simulink model "model"  (R2014a)
(part 4 of 4)

  L_186634762/LConn3 -- T_186634762__/RConn3 -- bus221/LConn1
  T_340152021__/RConn1 -- L_340152021/LConn1
  T_340152021__/RConn2 -- L_340152021/LConn2
  L_340152021/LConn3 -- T_340152021__/RConn3 -- bus222/LConn1
  T_265318415__/RConn1 -- L_265318415/LConn1
  T_265318415__/RConn2 -- L_265318415/LConn2
  L_265318415/LConn3 -- T_265318415__/RConn3 -- bus223/LConn1
  T_246972431__/RConn1 -- L_246972431/LConn1
  T_246972431__/RConn2 -- L_246972431/LConn2
  L_246972431/LConn3 -- T_246972431__/RConn3 -- bus224/LConn1
  T_234372891__/RConn1 -- L_234372891/LConn1
  T_234372891__/RConn2 -- L_234372891/LConn2
  L_234372891/LConn3 -- T_234372891__/RConn3 -- bus225/LConn1
  T_269492241__/RConn1 -- L_269492241/LConn1
  T_269492241__/RConn2 -- L_269492241/LConn2
  L_269492241/LConn3 -- T_269492241__/RConn3 -- bus226/LConn1
  T_160831508__/RConn1 -- L_160831508/LConn1
  T_160831508__/RConn2 -- L_160831508/LConn2
  L_160831508/LConn3 -- T_160831508__/RConn3 -- bus227/LConn1
  T_160831511__/RConn1 -- L_160831511/LConn1
  T_160831511__/RConn2 -- L_160831511/LConn2
  L_160831511/LConn3 -- T_160831511__/RConn3 -- bus228/LConn1
  T_399067566__/RConn1 -- L_399067566/LConn1
  T_399067566__/RConn2 -- L_399067566/LConn2
  L_399067566/LConn3 -- T_399067566__/RConn3 -- bus229/LConn1
  T_399067557__/RConn1 -- L_399067557/LConn1
  T_399067557__/RConn2 -- L_399067557/LConn2
  L_399067557/LConn3 -- T_399067557__/RConn3 -- bus230/LConn1
  T_167008794__/RConn1 -- L_167008794/LConn1
  T_167008794__/RConn2 -- L_167008794/LConn2
  L_167008794/LConn3 -- T_167008794__/RConn3 -- bus231/LConn1
  T_199476036__/RConn1 -- L_199476036/LConn1
  T_199476036__/RConn2 -- L_199476036/LConn2
  L_199476036/LConn3 -- T_199476036__/RConn3 -- bus232/LConn1
  T_311980589__Gardu_Induk_Alta_Prima/RConn1 -- L_311980589/LConn1
  T_311980589__Gardu_Induk_Alta_Prima/RConn2 -- L_311980589/LConn2
  L_311980589/LConn3 -- T_311980589__Gardu_Induk_Alta_Prima/RConn3 -- bus233/LConn1
  T_166644946__Gardu_Induk_Surabaya_Barat/RConn1 -- L_166644946/LConn1
  T_166644946__Gardu_Induk_Surabaya_Barat/RConn2 -- L_166644946/LConn2
  L_166644946/LConn3 -- T_166644946__Gardu_Induk_Surabaya_Barat/RConn3 -- bus234/LConn1
  T_277204741__/RConn1 -- L_277204741/LConn1
  T_277204741__/RConn2 -- L_277204741/LConn2
  L_277204741/LConn3 -- T_277204741__/RConn3 -- bus235/LConn1
  T_276990481__/RConn1 -- L_276990481/LConn1
  T_276990481__/RConn2 -- L_276990481/LConn2
  L_276990481/LConn3 -- T_276990481__/RConn3 -- bus236/LConn1
  T_228490272__Gardu_Induk_PLN_Palur/RConn1 -- L_228490272/LConn1
  T_228490272__Gardu_Induk_PLN_Palur/RConn2 -- L_228490272/LConn2
  L_228490272/LConn3 -- T_228490272__Gardu_Induk_PLN_Palur/RConn3 -- bus237/LConn1
  T_265030543__/RConn1 -- L_265030543/LConn1
  T_265030543__/RConn2 -- L_265030543/LConn2
  L_265030543/LConn3 -- T_265030543__/RConn3 -- bus238/LConn1
  T_268865917__/RConn1 -- L_268865917/LConn1
  T_268865917__/RConn2 -- L_268865917/LConn2
  L_268865917/LConn3 -- T_268865917__/RConn3 -- bus239/LConn1
  T_104412357__/RConn1 -- L_104412357/LConn1
  T_104412357__/RConn2 -- L_104412357/LConn2
  L_104412357/LConn3 -- T_104412357__/RConn3 -- bus240/LConn1
  T_311479841__Gardu_Sekar_Bungu/RConn1 -- L_311479841/LConn1
  T_311479841__Gardu_Sekar_Bungu/RConn2 -- L_311479841/LConn2
  L_311479841/LConn3 -- T_311479841__Gardu_Sekar_Bungu/RConn3 -- bus241/LConn1
  T_311666431__Gardu_Induk_Gili_Timur/RConn1 -- L_311666431/LConn1
  T_311666431__Gardu_Induk_Gili_Timur/RConn2 -- L_311666431/LConn2
  L_311666431/LConn3 -- T_311666431__Gardu_Induk_Gili_Timur/RConn3 -- bus242/LConn1
  T_311666430__Gardu_Induk_Bangkalan/RConn1 -- L_311666430/LConn1
  T_311666430__Gardu_Induk_Bangkalan/RConn2 -- L_311666430/LConn2
  L_311666430/LConn3 -- T_311666430__Gardu_Induk_Bangkalan/RConn3 -- bus243/LConn1
  T_398909637__/RConn1 -- L_398909637/LConn1
  T_398909637__/RConn2 -- L_398909637/LConn2
  L_398909637/LConn3 -- T_398909637__/RConn3 -- bus244/LConn1
  T_311485046__Gardu_Induk_Cerme/RConn1 -- L_311485046/LConn1
  T_311485046__Gardu_Induk_Cerme/RConn2 -- L_311485046/LConn2
  L_311485046/LConn3 -- T_311485046__Gardu_Induk_Cerme/RConn3 -- bus245/LConn1
  T_264855643__/RConn1 -- L_264855643/LConn1
  T_264855643__/RConn2 -- L_264855643/LConn2
  L_264855643/LConn3 -- T_264855643__/RConn3 -- bus246/LConn1
  T_265002737__/RConn1 -- L_265002737/LConn1
  T_265002737__/RConn2 -- L_265002737/LConn2
  L_265002737/LConn3 -- T_265002737__/RConn3 -- bus247/LConn1
  T_264855645__/RConn1 -- L_264855645/LConn1
  T_264855645__/RConn2 -- L_264855645/LConn2
  L_264855645/LConn3 -- T_264855645__/RConn3 -- bus248/LConn1
  T_248953893__/RConn1 -- L_248953893/LConn1
  T_248953893__/RConn2 -- L_248953893/LConn2
  L_248953893/LConn3 -- T_248953893__/RConn3 -- bus249/LConn1
  T_248953894__/RConn1 -- L_248953894/LConn1
  T_248953894__/RConn2 -- L_248953894/LConn2
  L_248953894/LConn3 -- T_248953894__/RConn3 -- bus250/LConn1
  T_267663602__/RConn1 -- L_267663602/LConn1
  T_267663602__/RConn2 -- L_267663602/LConn2
  L_267663602/LConn3 -- T_267663602__/RConn3 -- bus251/LConn1
  T_279284589__/RConn1 -- L_279284589/LConn1
  T_279284589__/RConn2 -- L_279284589/LConn2
  L_279284589/LConn3 -- T_279284589__/RConn3 -- bus252/LConn1
  T_195105324__/RConn1 -- L_195105324/LConn1
  T_195105324__/RConn2 -- L_195105324/LConn2
  L_195105324/LConn3 -- T_195105324__/RConn3 -- bus253/LConn1
  T_398925619__/RConn1 -- L_398925619/LConn1
  T_398925619__/RConn2 -- L_398925619/LConn2
  L_398925619/LConn3 -- T_398925619__/RConn3 -- bus254/LConn1
  T_195211467__/RConn1 -- L_195211467/LConn1
  T_195211467__/RConn2 -- L_195211467/LConn2
  L_195211467/LConn3 -- T_195211467__/RConn3 -- bus255/LConn1
  T_268846126__/RConn1 -- L_268846126/LConn1
  T_268846126__/RConn2 -- L_268846126/LConn2
  L_268846126/LConn3 -- T_268846126__/RConn3 -- bus256/LConn1
  T_268846115__/RConn1 -- L_268846115/LConn1
  T_268846115__/RConn2 -- L_268846115/LConn2
  L_268846115/LConn3 -- T_268846115__/RConn3 -- bus257/LConn1
  T_268831411__/RConn1 -- L_268831411/LConn1
  T_268831411__/RConn2 -- L_268831411/LConn2
  L_268831411/LConn3 -- T_268831411__/RConn3 -- bus258/LConn1
  T_399724591__/RConn1 -- L_399724591/LConn1
  T_399724591__/RConn2 -- L_399724591/LConn2
  L_399724591/LConn3 -- T_399724591__/RConn3 -- bus259/LConn1
  T_399724593__/RConn1 -- L_399724593/LConn1
  T_399724593__/RConn2 -- L_399724593/LConn2
  L_399724593/LConn3 -- T_399724593__/RConn3 -- bus260/LConn1
  T_162030133__/RConn1 -- L_162030133/LConn1
  T_162030133__/RConn2 -- L_162030133/LConn2
  L_162030133/LConn3 -- T_162030133__/RConn3 -- bus261/LConn1
  T_162030143__/RConn1 -- L_162030143/LConn1
  T_162030143__/RConn2 -- L_162030143/LConn2
  L_162030143/LConn3 -- T_162030143__/RConn3 -- bus262/LConn1
  T_162002076__/RConn1 -- L_162002076/LConn1
  T_162002076__/RConn2 -- L_162002076/LConn2
  L_162002076/LConn3 -- T_162002076__/RConn3 -- bus263/LConn1
  T_263932883__/RConn1 -- L_263932883/LConn1
  T_263932883__/RConn2 -- L_263932883/LConn2
  L_263932883/LConn3 -- T_263932883__/RConn3 -- bus264/LConn1
  T_311479840__Gardu_Induk_Segoromadu/RConn1 -- L_311479840/LConn1
  T_311479840__Gardu_Induk_Segoromadu/RConn2 -- L_311479840/LConn2
  L_311479840/LConn3 -- T_311479840__Gardu_Induk_Segoromadu/RConn3 -- bus265/LConn1
  T_311479839__Gardu_Induk_Petrokimia/RConn1 -- L_311479839/LConn1
  T_311479839__Gardu_Induk_Petrokimia/RConn2 -- L_311479839/LConn2
  L_311479839/LConn3 -- T_311479839__Gardu_Induk_Petrokimia/RConn3 -- bus266/LConn1
  T_398909625__/RConn1 -- L_398909625/LConn1
  T_398909625__/RConn2 -- L_398909625/LConn2
  L_398909625/LConn3 -- T_398909625__/RConn3 -- bus267/LConn1
  T_161951304__/RConn1 -- L_161951304/LConn1
  T_161951304__/RConn2 -- L_161951304/LConn2
  L_161951304/LConn3 -- T_161951304__/RConn3 -- bus268/LConn1
  T_399038176__/RConn1 -- L_399038176/LConn1
  T_399038176__/RConn2 -- L_399038176/LConn2
  L_399038176/LConn3 -- T_399038176__/RConn3 -- bus269/LConn1
  T_399038175__/RConn1 -- L_399038175/LConn1
  T_399038175__/RConn2 -- L_399038175/LConn2
  L_399038175/LConn3 -- T_399038175__/RConn3 -- bus270/LConn1
  T_161948635__/RConn1 -- L_161948635/LConn1
  T_161948635__/RConn2 -- L_161948635/LConn2
  L_161948635/LConn3 -- T_161948635__/RConn3 -- bus271/LConn1
  T_264713279__/RConn1 -- L_264713279/LConn1
  T_264713279__/RConn2 -- L_264713279/LConn2
  L_264713279/LConn3 -- T_264713279__/RConn3 -- bus272/LConn1
  T_269129296__/RConn1 -- L_269129296/LConn1
  T_269129296__/RConn2 -- L_269129296/LConn2
  L_269129296/LConn3 -- T_269129296__/RConn3 -- bus273/LConn1
  T_399067568__/RConn1 -- L_399067568/LConn1
  T_399067568__/RConn2 -- L_399067568/LConn2
  L_399067568/LConn3 -- T_399067568__/RConn3 -- bus274/LConn1
  T_265923575__/RConn1 -- L_265923575/LConn1
  T_265923575__/RConn2 -- L_265923575/LConn2
  L_265923575/LConn3 -- T_265923575__/RConn3 -- bus275/LConn1
  T_269468436__Gardu_Induk_PT__PLN/RConn1 -- L_269468436/LConn1
  T_269468436__Gardu_Induk_PT__PLN/RConn2 -- L_269468436/LConn2
  L_269468436/LConn3 -- T_269468436__Gardu_Induk_PT__PLN/RConn3 -- bus276/LConn1
  T_166632018__/RConn1 -- L_166632018/LConn1
  T_166632018__/RConn2 -- L_166632018/LConn2
  L_166632018/LConn3 -- T_166632018__/RConn3 -- bus277/LConn1
  T_104440761__/RConn1 -- L_104440761/LConn1
  T_104440761__/RConn2 -- L_104440761/LConn2
  L_104440761/LConn3 -- T_104440761__/RConn3 -- bus278/LConn1
  T_270800486__/RConn1 -- L_270800486/LConn1
  T_270800486__/RConn2 -- L_270800486/LConn2
  L_270800486/LConn3 -- T_270800486__/RConn3 -- bus279/LConn1
  T_265568004__/RConn1 -- L_265568004/LConn1
  T_265568004__/RConn2 -- L_265568004/LConn2
  L_265568004/LConn3 -- T_265568004__/RConn3 -- bus280/LConn1
  T_104538467__/RConn1 -- L_104538467/LConn1
  T_104538467__/RConn2 -- L_104538467/LConn2
  L_104538467/LConn3 -- T_104538467__/RConn3 -- bus281/LConn1
  T_269475415__/RConn1 -- L_269475415/LConn1
  T_269475415__/RConn2 -- L_269475415/LConn2
  L_269475415/LConn3 -- T_269475415__/RConn3 -- bus282/LConn1
  T_399067565__/RConn1 -- L_399067565/LConn1
  T_399067565__/RConn2 -- L_399067565/LConn2
  L_399067565/LConn3 -- T_399067565__/RConn3 -- bus283/LConn1
  T_269490141__/RConn1 -- L_269490141/LConn1
  T_269490141__/RConn2 -- L_269490141/LConn2
  L_269490141/LConn3 -- T_269490141__/RConn3 -- bus284/LConn1
  T_269490147__/RConn1 -- L_269490147/LConn1
  T_269490147__/RConn2 -- L_269490147/LConn2
  L_269490147/LConn3 -- T_269490147__/RConn3 -- bus285/LConn1
  T_269129304__/RConn1 -- L_269129304/LConn1
  T_269129304__/RConn2 -- L_269129304/LConn2
  L_269129304/LConn3 -- T_269129304__/RConn3 -- bus286/LConn1
  T_264410228__/RConn1 -- L_264410228/LConn1
  T_264410228__/RConn2 -- L_264410228/LConn2
  L_264410228/LConn3 -- T_264410228__/RConn3 -- bus287/LConn1
  T_265903214__/RConn1 -- L_265903214/LConn1
  T_265903214__/RConn2 -- L_265903214/LConn2
  L_265903214/LConn3 -- T_265903214__/RConn3 -- bus288/LConn1
  T_104412331__/RConn1 -- L_104412331/LConn1
  T_104412331__/RConn2 -- L_104412331/LConn2
  L_104412331/LConn3 -- T_104412331__/RConn3 -- bus289/LConn1
  T_265903215__/RConn1 -- L_265903215/LConn1
  T_265903215__/RConn2 -- L_265903215/LConn2
  L_265903215/LConn3 -- T_265903215__/RConn3 -- bus290/LConn1
  T_265588689__/RConn1 -- L_265588689/LConn1
  T_265588689__/RConn2 -- L_265588689/LConn2
  L_265588689/LConn3 -- T_265588689__/RConn3 -- bus291/LConn1
  T_121677176__Gardu_PLN_150KV_Banteng/RConn1 -- L_121677176/LConn1
  T_121677176__Gardu_PLN_150KV_Banteng/RConn2 -- L_121677176/LConn2
  L_121677176/LConn3 -- T_121677176__Gardu_PLN_150KV_Banteng/RConn3 -- bus292/LConn1
  T_399022980__/RConn1 -- L_399022980/LConn1
  T_399022980__/RConn2 -- L_399022980/LConn2
  L_399022980/LConn3 -- T_399022980__/RConn3 -- bus293/LConn1
  T_271376043__/RConn1 -- L_271376043/LConn1
  T_271376043__/RConn2 -- L_271376043/LConn2
  L_271376043/LConn3 -- T_271376043__/RConn3 -- bus294/LConn1
  T_268831422__/RConn1 -- L_268831422/LConn1
  T_268831422__/RConn2 -- L_268831422/LConn2
  L_268831422/LConn3 -- T_268831422__/RConn3 -- bus295/LConn1
  T_161980511__/RConn1 -- L_161980511/LConn1
  T_161980511__/RConn2 -- L_161980511/LConn2
  L_161980511/LConn3 -- T_161980511__/RConn3 -- bus296/LConn1
  T_161980518__/RConn1 -- L_161980518/LConn1
  T_161980518__/RConn2 -- L_161980518/LConn2
  L_161980518/LConn3 -- T_161980518__/RConn3 -- bus297/LConn1
  T_265903200__/RConn1 -- L_265903200/LConn1
  T_265903200__/RConn2 -- L_265903200/LConn2
  L_265903200/LConn3 -- T_265903200__/RConn3 -- bus298/LConn1
  T_277204263__/RConn1 -- L_277204263/LConn1
  T_277204263__/RConn2 -- L_277204263/LConn2
  L_277204263/LConn3 -- T_277204263__/RConn3 -- bus299/LConn1
  T_340205049__/RConn1 -- L_340205049/LConn1
  T_340205049__/RConn2 -- L_340205049/LConn2
  L_340205049/LConn3 -- T_340205049__/RConn3 -- bus300/LConn1
  T_268532906__/RConn1 -- L_268532906/LConn1
  T_268532906__/RConn2 -- L_268532906/LConn2
  L_268532906/LConn3 -- T_268532906__/RConn3 -- bus301/LConn1
  T_269129291__/RConn1 -- L_269129291/LConn1
  T_269129291__/RConn2 -- L_269129291/LConn2
  L_269129291/LConn3 -- T_269129291__/RConn3 -- bus302/LConn1
  T_339802233__/RConn1 -- L_339802233/LConn1
  T_339802233__/RConn2 -- L_339802233/LConn2
  L_339802233/LConn3 -- T_339802233__/RConn3 -- bus303/LConn1
  T_192989828__/RConn1 -- L_192989828/LConn1
  T_192989828__/RConn2 -- L_192989828/LConn2
  L_192989828/LConn3 -- T_192989828__/RConn3 -- bus304/LConn1
  T_339792684__/RConn1 -- L_339792684/LConn1
  T_339792684__/RConn2 -- L_339792684/LConn2
  L_339792684/LConn3 -- T_339792684__/RConn3 -- bus305/LConn1
  T_339796954__/RConn1 -- L_339796954/LConn1
  T_339796954__/RConn2 -- L_339796954/LConn2
  L_339796954/LConn3 -- T_339796954__/RConn3 -- bus306/LConn1
  T_340935922__/RConn1 -- L_340935922/LConn1
  T_340935922__/RConn2 -- L_340935922/LConn2
  L_340935922/LConn3 -- T_340935922__/RConn3 -- bus307/LConn1
  T_340963798__/RConn1 -- L_340963798/LConn1
  T_340963798__/RConn2 -- L_340963798/LConn2
  L_340963798/LConn3 -- T_340963798__/RConn3 -- bus308/LConn1
  T_311940754__Gardu_Induk_Krembangan/RConn1 -- L_311940754/LConn1
  T_311940754__Gardu_Induk_Krembangan/RConn2 -- L_311940754/LConn2
  L_311940754/LConn3 -- T_311940754__Gardu_Induk_Krembangan/RConn3 -- bus309/LConn1
  T_311942142__Gardu_Induk_Tandes/RConn1 -- L_311942142/LConn1
  T_311942142__Gardu_Induk_Tandes/RConn2 -- L_311942142/LConn2
  L_311942142/LConn3 -- T_311942142__Gardu_Induk_Tandes/RConn3 -- bus310/LConn1
  T_267968147__/RConn1 -- L_267968147/LConn1
  T_267968147__/RConn2 -- L_267968147/LConn2
  L_267968147/LConn3 -- T_267968147__/RConn3 -- bus311/LConn1
  T_269160480__/RConn1 -- L_269160480/LConn1
  T_269160480__/RConn2 -- L_269160480/LConn2
  L_269160480/LConn3 -- T_269160480__/RConn3 -- bus312/LConn1
  T_161948309__/RConn1 -- L_161948309/LConn1
  T_161948309__/RConn2 -- L_161948309/LConn2
  L_161948309/LConn3 -- T_161948309__/RConn3 -- bus313/LConn1
  T_161948315__/RConn1 -- L_161948315/LConn1
  T_161948315__/RConn2 -- L_161948315/LConn2
  L_161948315/LConn3 -- T_161948315__/RConn3 -- bus314/LConn1
  T_116023446__/RConn1 -- L_116023446/LConn1
  T_116023446__/RConn2 -- L_116023446/LConn2
  L_116023446/LConn3 -- T_116023446__/RConn3 -- bus315/LConn1
  T_229039262__/RConn1 -- L_229039262/LConn1
  T_229039262__/RConn2 -- L_229039262/LConn2
  L_229039262/LConn3 -- T_229039262__/RConn3 -- bus316/LConn1
  T_116023450__/RConn1 -- L_116023450/LConn1
  T_116023450__/RConn2 -- L_116023450/LConn2
  L_116023450/LConn3 -- T_116023450__/RConn3 -- bus317/LConn1
  T_399505626__/RConn1 -- L_399505626/LConn1
  T_399505626__/RConn2 -- L_399505626/LConn2
  L_399505626/LConn3 -- T_399505626__/RConn3 -- bus318/LConn1
  T_399505633__/RConn1 -- L_399505633/LConn1
  T_399505633__/RConn2 -- L_399505633/LConn2
  L_399505633/LConn3 -- T_399505633__/RConn3 -- bus319/LConn1
  T_399038179__/RConn1 -- L_399038179/LConn1
  T_399038179__/RConn2 -- L_399038179/LConn2
  L_399038179/LConn3 -- T_399038179__/RConn3 -- bus320/LConn1
  T_311432987__Gardu_Induk_Kenjeran/RConn1 -- L_311432987/LConn1
  T_311432987__Gardu_Induk_Kenjeran/RConn2 -- L_311432987/LConn2
  L_311432987/LConn3 -- T_311432987__Gardu_Induk_Kenjeran/RConn3 -- bus321/LConn1
  T_311432989__Gardu_Induk_Sukolilo/RConn1 -- L_311432989/LConn1
  T_311432989__Gardu_Induk_Sukolilo/RConn2 -- L_311432989/LConn2
  L_311432989/LConn3 -- T_311432989__Gardu_Induk_Sukolilo/RConn3 -- bus322/LConn1
  T_311432990__Gardu_Induk_Ujung/RConn1 -- L_311432990/LConn1
  T_311432990__Gardu_Induk_Ujung/RConn2 -- L_311432990/LConn2
  L_311432990/LConn3 -- T_311432990__Gardu_Induk_Ujung/RConn3 -- bus323/LConn1
  T_311957671__Gardu_Induk_Gondang_Wetan/RConn1 -- L_311957671/LConn1
  T_311957671__Gardu_Induk_Gondang_Wetan/RConn2 -- L_311957671/LConn2
  L_311957671/LConn3 -- T_311957671__Gardu_Induk_Gondang_Wetan/RConn3 -- bus324/LConn1
  T_340947951__/RConn1 -- L_340947951/LConn1
  T_340947951__/RConn2 -- L_340947951/LConn2
  L_340947951/LConn3 -- T_340947951__/RConn3 -- bus325/LConn1
  T_399057180__/RConn1 -- L_399057180/LConn1
  T_399057180__/RConn2 -- L_399057180/LConn2
  L_399057180/LConn3 -- T_399057180__/RConn3 -- bus326/LConn1
  T_199476032__/RConn1 -- L_199476032/LConn1
  T_199476032__/RConn2 -- L_199476032/LConn2
  L_199476032/LConn3 -- T_199476032__/RConn3 -- bus327/LConn1
  T_161969969__/RConn1 -- L_161969969/LConn1
  T_161969969__/RConn2 -- L_161969969/LConn2
  L_161969969/LConn3 -- T_161969969__/RConn3 -- bus328/LConn1
  T_265030533__/RConn1 -- L_265030533/LConn1
  T_265030533__/RConn2 -- L_265030533/LConn2
  L_265030533/LConn3 -- T_265030533__/RConn3 -- bus329/LConn1
  T_182845612__/RConn1 -- L_182845612/LConn1
  T_182845612__/RConn2 -- L_182845612/LConn2
  L_182845612/LConn3 -- T_182845612__/RConn3 -- bus330/LConn1
  T_272989134__/RConn1 -- L_272989134/LConn1
  T_272989134__/RConn2 -- L_272989134/LConn2
  L_272989134/LConn3 -- T_272989134__/RConn3 -- bus331/LConn1
  T_311432988__Gardu_Induk_Rungkut/RConn1 -- L_311432988/LConn1
  T_311432988__Gardu_Induk_Rungkut/RConn2 -- L_311432988/LConn2
  L_311432988/LConn3 -- T_311432988__Gardu_Induk_Rungkut/RConn3 -- bus332/LConn1
  T_189064370__Gardu_Induk_Situbondo_(PLN)/RConn1 -- L_189064370/LConn1
  T_189064370__Gardu_Induk_Situbondo_(PLN)/RConn2 -- L_189064370/LConn2
  L_189064370/LConn3 -- T_189064370__Gardu_Induk_Situbondo_(PLN)/RConn3 -- bus333/LConn1
  T_398892599__/RConn1 -- L_398892599/LConn1
  T_398892599__/RConn2 -- L_398892599/LConn2
  L_398892599/LConn3 -- T_398892599__/RConn3 -- bus334/LConn1
  T_186337693__Gardu_Induk_Banyuwangi/RConn1 -- L_186337693/LConn1
  T_186337693__Gardu_Induk_Banyuwangi/RConn2 -- L_186337693/LConn2
  L_186337693/LConn3 -- T_186337693__Gardu_Induk_Banyuwangi/RConn3 -- bus335/LConn1
  T_339796951__/RConn1 -- L_339796951/LConn1
  T_339796951__/RConn2 -- L_339796951/LConn2
  L_339796951/LConn3 -- T_339796951__/RConn3 -- bus336/LConn1
  T_268865913__/RConn1 -- L_268865913/LConn1
  T_268865913__/RConn2 -- L_268865913/LConn2
  L_268865913/LConn3 -- T_268865913__/RConn3 -- bus337/LConn1
  T_399714486__/RConn1 -- L_399714486/LConn1
  T_399714486__/RConn2 -- L_399714486/LConn2
  L_399714486/LConn3 -- T_399714486__/RConn3 -- bus338/LConn1
  T_257725651__/RConn1 -- L_257725651/LConn1
  T_257725651__/RConn2 -- L_257725651/LConn2
  L_257725651/LConn3 -- T_257725651__/RConn3 -- bus339/LConn1
  T_244815736__/RConn1 -- L_244815736/LConn1
  T_244815736__/RConn2 -- L_244815736/LConn2
  L_244815736/LConn3 -- T_244815736__/RConn3 -- bus340/LConn1
  T_157804728__/RConn1 -- L_157804728/LConn1
  T_157804728__/RConn2 -- L_157804728/LConn2
  L_157804728/LConn3 -- T_157804728__/RConn3 -- bus341/LConn1
  T_198149824_500000_Gardu_Listrik/RConn1 -- L_198149824/LConn1
  T_198149824_500000_Gardu_Listrik/RConn2 -- L_198149824/LConn2
  L_198149824/LConn3 -- T_198149824_500000_Gardu_Listrik/RConn3 -- bus342/LConn1
  T_249207412__/RConn1 -- L_249207412/LConn1
  T_249207412__/RConn2 -- L_249207412/LConn2
  L_249207412/LConn3 -- T_249207412__/RConn3 -- bus343/LConn1
  T_277204262__/RConn1 -- L_277204262/LConn1
  T_277204262__/RConn2 -- L_277204262/LConn2
  L_277204262/LConn3 -- T_277204262__/RConn3 -- bus344/LConn1
  T_261184996__/RConn1 -- L_261184996/LConn1
  T_261184996__/RConn2 -- L_261184996/LConn2
  L_261184996/LConn3 -- T_261184996__/RConn3 -- bus345/LConn1
  T_398909635__/RConn1 -- L_398909635/LConn1
  T_398909635__/RConn2 -- L_398909635/LConn2
  L_398909635/LConn3 -- T_398909635__/RConn3 -- bus346/LConn1
  T_352100214__/RConn1 -- L_352100214/LConn1
  T_352100214__/RConn2 -- L_352100214/LConn2
  L_352100214/LConn3 -- T_352100214__/RConn3 -- bus347/LConn1
  T_166699717__/RConn1 -- L_166699717/LConn1
  T_166699717__/RConn2 -- L_166699717/LConn2
  L_166699717/LConn3 -- T_166699717__/RConn3 -- bus348/LConn1
  T_339792673__/RConn1 -- L_339792673/LConn1
  T_339792673__/RConn2 -- L_339792673/LConn2
  L_339792673/LConn3 -- T_339792673__/RConn3 -- bus349/LConn1
  T_258997962__Gardu_Induk_PLN/RConn1 -- L_258997962/LConn1
  T_258997962__Gardu_Induk_PLN/RConn2 -- L_258997962/LConn2
  L_258997962/LConn3 -- T_258997962__Gardu_Induk_PLN/RConn3 -- bus350/LConn1
  T_340978671__/RConn1 -- L_340978671/LConn1
  T_340978671__/RConn2 -- L_340978671/LConn2
  L_340978671/LConn3 -- T_340978671__/RConn3 -- bus351/LConn1
  T_311963425__Gardu_Induk_Darmo_Grande/RConn1 -- L_311963425/LConn1
  T_311963425__Gardu_Induk_Darmo_Grande/RConn2 -- L_311963425/LConn2
  L_311963425/LConn3 -- T_311963425__Gardu_Induk_Darmo_Grande/RConn3 -- bus352/LConn1
  T_311963427__Gardu_Induk_Karang_Pilang/RConn1 -- L_311963427/LConn1
  T_311963427__Gardu_Induk_Karang_Pilang/RConn2 -- L_311963427/LConn2
  L_311963427/LConn3 -- T_311963427__Gardu_Induk_Karang_Pilang/RConn3 -- bus353/LConn1
  T_398787876__/RConn1 -- L_398787876/LConn1
  T_398787876__/RConn2 -- L_398787876/LConn2
  L_398787876/LConn3 -- T_398787876__/RConn3 -- bus354/LConn1
  T_309311292__Gardu_Induk_Lamreung/RConn1 -- L_309311292/LConn1
  T_309311292__Gardu_Induk_Lamreung/RConn2 -- L_309311292/LConn2
  L_309311292/LConn3 -- T_309311292__Gardu_Induk_Lamreung/RConn3 -- bus355/LConn1
  T_161963229__/RConn1 -- L_161963229/LConn1
  T_161963229__/RConn2 -- L_161963229/LConn2
  L_161963229/LConn3 -- T_161963229__/RConn3 -- bus356/LConn1
  T_252566435__GARDU_INDUK_PLN/RConn1 -- L_252566435/LConn1
  T_252566435__GARDU_INDUK_PLN/RConn2 -- L_252566435/LConn2
  L_252566435/LConn3 -- T_252566435__GARDU_INDUK_PLN/RConn3 -- bus357/LConn1
  T_277183760__/RConn1 -- L_277183760/LConn1
  T_277183760__/RConn2 -- L_277183760/LConn2
  L_277183760/LConn3 -- T_277183760__/RConn3 -- bus358/LConn1
  T_265002738__/RConn1 -- L_265002738/LConn1
  T_265002738__/RConn2 -- L_265002738/LConn2
  L_265002738/LConn3 -- T_265002738__/RConn3 -- bus359/LConn1
  T_265002740__/RConn1 -- L_265002740/LConn1
  T_265002740__/RConn2 -- L_265002740/LConn2
  L_265002740/LConn3 -- T_265002740__/RConn3 -- bus360/LConn1
  T_311666433__Gardu_Induk_Sampang/RConn1 -- L_311666433/LConn1
  T_311666433__Gardu_Induk_Sampang/RConn2 -- L_311666433/LConn2
  L_311666433/LConn3 -- T_311666433__Gardu_Induk_Sampang/RConn3 -- bus361/LConn1
  T_311666432__Gardu_Induk_Pamekasan/RConn1 -- L_311666432/LConn1
  T_311666432__Gardu_Induk_Pamekasan/RConn2 -- L_311666432/LConn2
  L_311666432/LConn3 -- T_311666432__Gardu_Induk_Pamekasan/RConn3 -- bus362/LConn1
  T_311666434__Gardu_Induk_Sumenep/RConn1 -- L_311666434/LConn1
  T_311666434__Gardu_Induk_Sumenep/RConn2 -- L_311666434/LConn2
  L_311666434/LConn3 -- T_311666434__Gardu_Induk_Sumenep/RConn3 -- bus363/LConn1
  T_153303534__PLT/RConn1 -- L_153303534/LConn1
  T_153303534__PLT/RConn2 -- L_153303534/LConn2
  L_153303534/LConn3 -- T_153303534__PLT/RConn3 -- bus364/LConn1
  T_399057165__/RConn1 -- L_399057165/LConn1
  T_399057165__/RConn2 -- L_399057165/LConn2
  L_399057165/LConn3 -- T_399057165__/RConn3 -- bus365/LConn1
  T_264106354__/RConn1 -- L_264106354/LConn1
  T_264106354__/RConn2 -- L_264106354/LConn2
  L_264106354/LConn3 -- T_264106354__/RConn3 -- bus366/LConn1
  T_277204260__/RConn1 -- L_277204260/LConn1
  T_277204260__/RConn2 -- L_277204260/LConn2
  L_277204260/LConn3 -- T_277204260__/RConn3 -- bus367/LConn1
  T_277183761__/RConn1 -- L_277183761/LConn1
  T_277183761__/RConn2 -- L_277183761/LConn2
  L_277183761/LConn3 -- T_277183761__/RConn3 -- bus368/LConn1
  T_271678852__/RConn1 -- L_271678852/LConn1
  T_271678852__/RConn2 -- L_271678852/LConn2
  L_271678852/LConn3 -- T_271678852__/RConn3 -- bus369/LConn1
  T_119360808__Gardu_Induk_Wonorejo/RConn1 -- L_119360808/LConn1
  T_119360808__Gardu_Induk_Wonorejo/RConn2 -- L_119360808/LConn2
  L_119360808/LConn3 -- T_119360808__Gardu_Induk_Wonorejo/RConn3 -- bus370/LConn1
  T_339792680__/RConn1 -- L_339792680/LConn1
  T_339792680__/RConn2 -- L_339792680/LConn2
  L_339792680/LConn3 -- T_339792680__/RConn3 -- bus371/LConn1
  T_185683916__/RConn1 -- L_185683916/LConn1
  T_185683916__/RConn2 -- L_185683916/LConn2
  L_185683916/LConn3 -- T_185683916__/RConn3 -- bus372/LConn1
  T_339792685__/RConn1 -- L_339792685/LConn1
  T_339792685__/RConn2 -- L_339792685/LConn2
  L_339792685/LConn3 -- T_339792685__/RConn3 -- bus373/LConn1
  T_398972213__/RConn1 -- L_398972213/LConn1
  T_398972213__/RConn2 -- L_398972213/LConn2
  L_398972213/LConn3 -- T_398972213__/RConn3 -- bus374/LConn1
  T_265030532__/RConn1 -- L_265030532/LConn1
  T_265030532__/RConn2 -- L_265030532/LConn2
  L_265030532/LConn3 -- T_265030532__/RConn3 -- bus375/LConn1
  T_265030541__/RConn1 -- L_265030541/LConn1
  T_265030541__/RConn2 -- L_265030541/LConn2
  L_265030541/LConn3 -- T_265030541__/RConn3 -- bus376/LConn1
  T_340978685__/RConn1 -- L_340978685/LConn1
  T_340978685__/RConn2 -- L_340978685/LConn2
  L_340978685/LConn3 -- T_340978685__/RConn3 -- bus377/LConn1
  T_271991718__Gardu_Induk_Indonesia_Power/RConn1 -- L_271991718/LConn1
  T_271991718__Gardu_Induk_Indonesia_Power/RConn2 -- L_271991718/LConn2
  L_271991718/LConn3 -- T_271991718__Gardu_Induk_Indonesia_Power/RConn3 -- bus378/LConn1
  T_253654957__/RConn1 -- L_253654957/LConn1
  T_253654957__/RConn2 -- L_253654957/LConn2
  L_253654957/LConn3 -- T_253654957__/RConn3 -- bus379/LConn1
  T_261185003__/RConn1 -- L_261185003/LConn1
  T_261185003__/RConn2 -- L_261185003/LConn2
  L_261185003/LConn3 -- T_261185003__/RConn3 -- bus380/LConn1
  T_399094735__/RConn1 -- L_399094735/LConn1
  T_399094735__/RConn2 -- L_399094735/LConn2
  L_399094735/LConn3 -- T_399094735__/RConn3 -- bus381/LConn1
  T_269490135__/RConn1 -- L_269490135/LConn1
  T_269490135__/RConn2 -- L_269490135/LConn2
  L_269490135/LConn3 -- T_269490135__/RConn3 -- bus382/LConn1
  T_398909640__/RConn1 -- L_398909640/LConn1
  T_398909640__/RConn2 -- L_398909640/LConn2
  L_398909640/LConn3 -- T_398909640__/RConn3 -- bus383/LConn1
  T_399100034__/RConn1 -- L_399100034/LConn1
  T_399100034__/RConn2 -- L_399100034/LConn2
  L_399100034/LConn3 -- T_399100034__/RConn3 -- bus384/LConn1
  T_399100035__/RConn1 -- L_399100035/LConn1
  T_399100035__/RConn2 -- L_399100035/LConn2
  L_399100035/LConn3 -- T_399100035__/RConn3 -- bus385/LConn1
  T_399022979__/RConn1 -- L_399022979/LConn1
  T_399022979__/RConn2 -- L_399022979/LConn2
  L_399022979/LConn3 -- T_399022979__/RConn3 -- bus386/LConn1
  T_271376037__/RConn1 -- L_271376037/LConn1
  T_271376037__/RConn2 -- L_271376037/LConn2
  L_271376037/LConn3 -- T_271376037__/RConn3 -- bus387/LConn1
  T_264550744__/RConn1 -- L_264550744/LConn1
  T_264550744__/RConn2 -- L_264550744/LConn2
  L_264550744/LConn3 -- T_264550744__/RConn3 -- bus388/LConn1
  T_267626657__/RConn1 -- L_267626657/LConn1
  T_267626657__/RConn2 -- L_267626657/LConn2
  L_267626657/LConn3 -- T_267626657__/RConn3 -- bus389/LConn1
  T_199476040__/RConn1 -- L_199476040/LConn1
  T_199476040__/RConn2 -- L_199476040/LConn2
  L_199476040/LConn3 -- T_199476040__/RConn3 -- bus390/LConn1
  T_169444592__/RConn1 -- L_169444592/LConn1
  T_169444592__/RConn2 -- L_169444592/LConn2
  L_169444592/LConn3 -- T_169444592__/RConn3 -- bus391/LConn1
  T_264410236__/RConn1 -- L_264410236/LConn1
  T_264410236__/RConn2 -- L_264410236/LConn2
  L_264410236/LConn3 -- T_264410236__/RConn3 -- bus392/LConn1
  T_161960933__/RConn1 -- L_161960933/LConn1
  T_161960933__/RConn2 -- L_161960933/LConn2
  L_161960933/LConn3 -- T_161960933__/RConn3 -- bus393/LConn1
  T_399038181__/RConn1 -- L_399038181/LConn1
  T_399038181__/RConn2 -- L_399038181/LConn2
  L_399038181/LConn3 -- T_399038181__/RConn3 -- bus394/LConn1
